simulink model "realmodel_lqr_updown_v3_2016b"  (R2016b)
settings: Solver=ode45  StartTime=0.0  StopTime=10  RelTol=1e-3  EnableMultiTasking=on
InitFcn:
  | lin_discr_model_test
values from neighbouring files (symbols this model uses):
  A_eq3_d = sysd3.A    [lin_discr_model_test.m]
  B_eq3_d = sysd3.B    [lin_discr_model_test.m]
  C_eq3_d_n = sysd3_n.C    [lin_discr_model_test.m]
  D_eq3_d = sysd3.D    [lin_discr_model_test.m]
  Ts = 0.01    [lin_discr_model_test.m]
undefined symbols (not defined in the file or in its folder): adingain, adinoffs, daoutgain, daoutoffs, DiscIntNeverNeededParam, Discrete, K3_lq, Ki3, Time
undefined symbols (not defined in the file): h
libraries: ctrlSharedLib x1
settings Model: Creator=rbabuska  LastModifiedBy=jannekeblok
settings DataIOCC: LimitDataPoints=on  SaveFormat=Array  SignalLoggingName=sigsOut
settings OptimizationCC: BooleanDataType=off  ExpressionDepthLimit=2147483647  InitFltsAndDblsToZero=on  LifeSpan=inf
settings DebuggingCC: SaveWithParameterizedLinksMsg=none  SignalResolutionControl=TryResolveAllWithWarning  MultiTaskDSMMsg=warning  MultiTaskCondExecSysMsg=none  AllowSymbolicDim=off  StateNameClashWarn=warning  SFUnexpectedBacktrackingDiag=warning  SFNoUnconditionalDefaultTransitionDiag=warning  SFExecutionAtInitializationDiag=none
settings HardwareCC: ProdBitPerPointer=32  ProdBitPerSizeT=32  ProdBitPerPtrDiffT=32  ProdLargestAtomicFloat=None  ProdIntDivRoundTo=Undefined  ProdEndianess=Unspecified  ProdWordSize=32  ProdHWDeviceType=32-bit Generic  TargetUnknown=on
settings ModelReferenceCC: PropagateSignalLabelsOutOfModel=off
settings GRTTargetCC: TargetFcnLib=ansi_tfl_tmw.mat  TargetLangStandard=C89/C90 (ANSI)  GeneratePreprocessorConditionals=Disable all  CombineOutputUpdateFcns=off  GRTInterface=on
settings ConfigComp: CovMetricSettings=dw  CovHtmlReporting=on  CovSaveCumulativeToWorkspaceVar=on  CovSaveSingleToWorkspaceVar=on  CovExternalEMLEnable=off

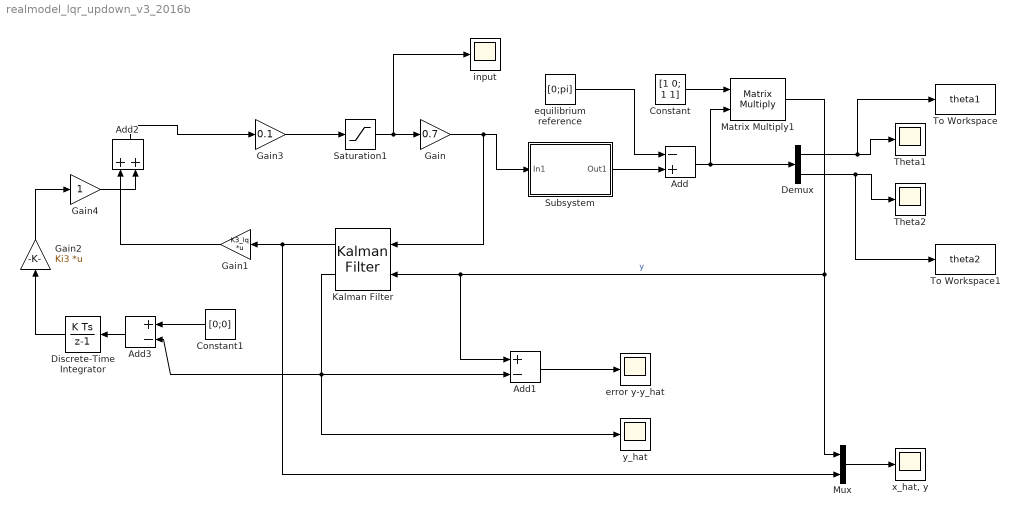
== system realmodel_lqr_updown_v3_2016b ==
  Add : Sum  Inputs=-+
  Add1 : Sum  Inputs=+-
  Add2 : Sum
  Add3 : Sum  Inputs=+-
  Constant : Constant  Value=[1 0; 1 1]
  Constant1 : Constant  Value=[0;0]  SampleTime=Ts
  Demux : Demux  Outputs=2
  Discrete-Time Integrator : DiscreteIntegrator  InitialConditionSetting=State (most efficient)  SampleTime=Ts  ICPrevOutput=DiscIntNeverNeededParam  ICPrevScaledInput=DiscIntNeverNeededParam
  Gain : Gain  Gain=0.7
  Gain1 : Gain  Gain=K3_lq  Multiplication=Matrix(K*u)
  Gain2 : Gain  Gain=Ki3  Multiplication=Matrix(K*u)
  Gain3 : Gain  Gain=0.1
  Gain4 : Gain
  Kalman Filter : ctrlSharedLib/Kalman Filter  TimeDomain=Discrete-Time  UseCurrentEstimator=on  ModelSource=Individual A, B, C, D matrices  ModelSourceVariable=ss(0.95,1,1,0,1)  A=A_eq3_d  B=B_eq3_d  C=C_eq3_d_n  D=D_eq3_d  NumberOfStates=1  NumberOfInputs=1  NumberOfOutputs=1  InitialEstimateSource=Dialog  X0=[0;0;0;0]  P0=10  UseK=off  UseGH=off  NumberOfProcessNoiseInputs=1  G=1  TimeInvariantG=on  H=0  TimeInvariantH=on  Q=diag([100 100 0.01 0.01])  TimeInvariantQ=on  R=0.00001  TimeInvariantR=on  N=0  TimeInvariantN=on  AddInputPort=on  AddEnablePort=off  OutputEstimatedY=on  OutputP=off  Ts=Ts
  Matrix Multiply1 : Product  Multiplication=Matrix(*)
  Mux : Mux  Inputs=2
  Saturation1 : Saturate  UpperLimit=1  LowerLimit=-1
  Subsystem : Subsystem
      mask Display: disp('Rotational\nPendulum')
  Theta1 : Scope
  Theta2 : Scope
  To Workspace : ToWorkspace  VariableName=theta1  SaveFormat=Timeseries  SampleTime=-1
  To Workspace1 : ToWorkspace  VariableName=theta2  SaveFormat=Timeseries  SampleTime=-1
  equilibrium reference : Constant  Value=[0;pi]  SampleTime=Ts
  error y-y_hat : Scope
  input : Scope
  "x_hat, y" : Scope
  y_hat : Scope
  wires:
  Demux/1 -> To Workspace/1, Theta1/1
  Demux/2 -> To Workspace1/1, Theta2/1
  equilibrium reference/1 -> Add/1
  Subsystem/1(Out1) -> Add/2
  Add/1 -> Matrix Multiply1/2, Demux/1
  Add1/1 -> error y-y_hat/1
  Saturation1/1 -> input/1, Gain/1
  Gain/1 -> Kalman Filter/1, Subsystem/1(In1)
  Constant/1 -> Matrix Multiply1/1
  Matrix Multiply1/1 -> Add1/1, Kalman Filter/2, Mux/1  "y"
  Mux/1 -> "x_hat, y"/1
  Gain1/1 -> Add2/1
  Constant1/1 -> Add3/1
  Add3/1 -> Discrete-Time Integrator/1
  Discrete-Time Integrator/1 -> Gain2/1
  Gain2/1 -> Gain4/1
  Add2/1 -> Gain3/1
  Gain4/1 -> Add2/2
  Gain3/1 -> Saturation1/1
  Kalman Filter/1 -> Mux/2, Gain1/1
  Kalman Filter/2 -> y_hat/1, Add1/2, Add3/2

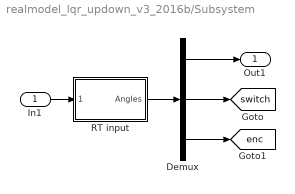
== system realmodel_lqr_updown_v3_2016b/Subsystem ==
  In1 : Inport
  Demux : Demux  Outputs=[2 4 1]
  RT input : Subsystem  mask{Ts=h, channels=[6 7]}
      mask prompts: Ts "Sample time [s]:"; channels "Channels to read (e.g., [6 7])"
      mask init:
      | hwinit;
      | 
      | % initialize FPGA
      | fugihandle = fugiboard('Open', 'Pendulum1');
      | fugihandle.WatchdogTimeout = 0.5;
      | fugiboard('SetParams', fugihandle);
      | fugiboard('Write', fugihandle, 0, 0, 0, 0);  % dummy write to sync interface board
      | fugiboard('Write', fugihandle, 5, 1, 0, 0);  % reset position, activate relay
      | data = fugiboard('Read', fugihandle);        % get version info from FPGA
      | % model = bitshift(data(1), -5); 
      | % version = bitand(data(1), 31);
      | % disp(sprintf('FPGA setup %d, version %d', model, version)); % for the B&P it should say 1 1, or else there is a problem
      | fugiboard('Write', fugihandle, 0, 1, 0, 0);  % end reset
      | pause(0.1);                         % give relay some time to respond
      mask Display: disp('Rotational\nPendulum')
  Out1 : Outport
  tag scope: enc=global, switch=global
  wires:
  RT input/1(Angles) -> Demux/1
  Demux/1 -> Out1/1
  Demux/2 -> [switch]
  Demux/3 -> [enc]
  In1/1 -> RT input/1(Motors)

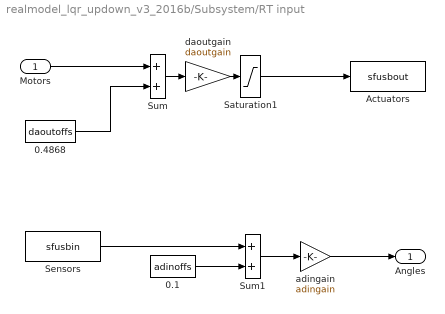
== system realmodel_lqr_updown_v3_2016b/Subsystem/RT input ==
  Motors : Inport
  0.1 : Constant  Value=adinoffs
  0.4868 : Constant  Value=daoutoffs
  Actuators : S-Function  FunctionName=sfusbout  Parameters=Ts, fugihandle  SFunctionDeploymentMode=off  EnableBusSupport=off
  Saturation1 : Saturate  UpperLimit=10  LowerLimit=-10
  Sensors : S-Function  FunctionName=sfusbin  Parameters=Ts, fugihandle, channels  SFunctionDeploymentMode=off  EnableBusSupport=off
  Sum : Sum  SaturateOnIntegerOverflow=on  InputSameDT=on  OutDataTypeStr=Inherit: Same as first input
  Sum1 : Sum  SaturateOnIntegerOverflow=on  InputSameDT=on  OutDataTypeStr=Inherit: Same as first input
  adingain : Gain  Gain=adingain  SaturateOnIntegerOverflow=on  OutDataTypeStr=Inherit: Same as input  ParamDataTypeStr=Inherit: Same as input
  daoutgain : Gain  Gain=daoutgain  SaturateOnIntegerOverflow=on  OutDataTypeStr=Inherit: Same as input  ParamDataTypeStr=Inherit: Same as input
  Angles : Outport
  wires:
  Sum/1 -> daoutgain/1
  0.4868/1 -> Sum/2
  Motors/1 -> Sum/1
  Sum1/1 -> adingain/1
  0.1/1 -> Sum1/2
  adingain/1 -> Angles/1
  Saturation1/1 -> Actuators/1
  daoutgain/1 -> Saturation1/1
  Sensors/1 -> Sum1/1
